simulink library "hfe_lib"  (Simulink 7.8)
settings: Solver=ode45  SolverMode=SingleTasking  StartTime=0.0  StopTime=10.0  RelTol=1e-3
values from neighbouring files (symbols this model uses):
  K_TACH = K_TACH_V2HZ * HZ2RPM    (= 1063.8)    [setup_hfe.m]
  K_TEMP = 20    [setup_hfe.m]
undefined symbols (not defined in the file or in its folder): HIL, qc_get_step_size
libraries: quarc_library x3
settings Model: Creator=MLevis  LastModifiedBy=pmartin  ExtModeTrigDuration=10000

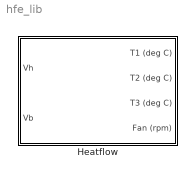
== system hfe_lib ==
  Heatflow : Subsystem

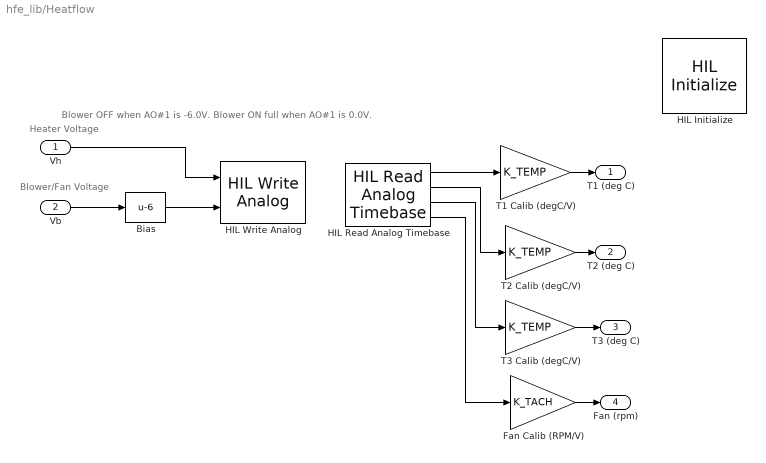
== system hfe_lib/Heatflow ==
  note: Blower OFF when AO#1 is -6.0V.
      | Blower ON full when AO#1 is 0.0V.
  note: Blower/Fan Voltage
  note: Heater Voltage
  Vh : Inport
  Vb : Inport  Port=2
  Bias : Bias  Bias=-6
  Fan Calib (RPM/V) : Gain  Gain=K_TACH
  HIL Initialize : quarc_library/Data Acquisition/Generic/Configuration/HIL Initialize  Priority=-99  object_name=HIL-1  board_type=q8_usb  board_number=0  board_options=update_rate=normal;decimation=1  exclusive=off  active=off  hardware_clocks=[0:2]  clock_modes=[]  initial_clock_frequencies=[]  set_clock_params_at_start=off  set_clock_params_at_switch_in=off  set_clock_frequencies_at_start=off  set_clock_frequencies_at_switch_in=off  analog_input_channels=[0:7]  analog_input_maximums=10  analog_input_minimums=-10  set_analog_input_params_at_start=on  set_analog_input_params_at_switch_in=off  analog_output_channels=[0:7]  analog_output_maximums=10  analog_output_minimums=-10  initial_analog_outputs=[0]  final_analog_outputs=[0]  watchdog_analog_outputs=0  set_analog_output_params_at_start=on  set_analog_output_params_at_switch_in=off  set_analog_outputs_at_start=on  set_analog_outputs_at_switch_in=off  set_analog_outputs_at_terminate=on  set_analog_outputs_at_switch_out=off  set_analog_outputs_on_watchdog=off  digital_input_channels=[]  digital_output_channels=[]  digital_output_configuration=[]  initial_digital_outputs=[1]  final_digital_outputs=[1]  watchdog_digital_outputs=[1]  set_digital_output_params_at_start=off  set_digital_output_params_at_switch_in=off  set_digital_outputs_at_start=on  set_digital_outputs_at_switch_in=off  set_digital_outputs_at_terminate=on  set_digital_outputs_at_switch_out=off  set_digital_outputs_on_watchdog=off  encoder_channels=[0:7]  quadrature=[4]  encoder_filter_frequency=[]  initial_encoder_counts=[0]  set_encoder_params_at_start=on  set_encoder_params_at_switch_in=off  set_encoder_counts_at_start=on  set_encoder_counts_at_switch_in=off  pwm_channels=[0:7]  pwm_modes=0  pwm_frequency=99.532799999999995e6/4095  pwm_configuration=[0]  pwm_alignment=[0]  pwm_polarity=[1]  pwm_leading_deadband=[0]  pwm_trailing_deadband=[0]  initial_pwm_outputs=[0]  final_pwm_outputs=[0]  watchdog_pwm_outputs=[0]  set_pwm_params_at_start=on  set_pwm_params_at_switch_in=off  set_pwm_outputs_at_start=on  set_pwm_outputs_at_switch_in=off  set_pwm_outputs_at_terminate=on  set_pwm_outputs_at_switch_out=off  set_pwm_outputs_on_watchdog=off  other_output_channels=[]  initial_other_outputs=[]  final_other_outputs=[]  watchdog_other_outputs=[]  set_other_outputs_at_start=off  set_other_outputs_at_switch_in=off  set_other_outputs_at_terminate=off  set_other_outputs_at_switch_out=off  set_other_outputs_on_watchdog=off
  HIL Read Analog Timebase : quarc_library/Data Acquisition/Generic/Timebases/HIL Read Analog Timebase  object_name=HIL-1  clock=0  channels=[0:3]  samples_in_buffer=max(ceil(1/qc_get_step_size), 1)  active=on  vector_output=off
      settings: AttributesFormatString=(%<object_name>)
  HIL Write Analog : quarc_library/Data Acquisition/Generic/Immediate I//O/HIL Write Analog  object_name=HIL-1  channels=[0,1]  sample_time=-1  active=off  vector_input=off
  T1 Calib (degC/V) : Gain  Gain=K_TEMP
  T2 Calib (degC/V) : Gain  Gain=K_TEMP
  T3 Calib (degC/V) : Gain  Gain=K_TEMP
  T1 (deg C) : Outport
  T2 (deg C) : Outport  Port=2
  T3 (deg C) : Outport  Port=3
  Fan (rpm) : Outport  Port=4
  wires:
  Bias/1 -> HIL Write Analog/2
  Fan Calib (RPM/V)/1 -> Fan (rpm)/1
  T1 Calib (degC/V)/1 -> T1 (deg C)/1
  HIL Read Analog Timebase/1 -> T1 Calib (degC/V)/1
  HIL Read Analog Timebase/2 -> T2 Calib (degC/V)/1
  HIL Read Analog Timebase/3 -> T3 Calib (degC/V)/1
  Vb/1 -> Bias/1
  HIL Read Analog Timebase/4 -> Fan Calib (RPM/V)/1
  Vh/1 -> HIL Write Analog/1
  T2 Calib (degC/V)/1 -> T2 (deg C)/1
  T3 Calib (degC/V)/1 -> T3 (deg C)/1
